simulink library "Normalization"  (R2014b)
settings: Solver=ode45  StartTime=0.0  StopTime=10.0  RelTol=1e-3
libraries: DivisionVectorScalar x1
settings Model: Creator=Hp  LastModifiedBy=Hp

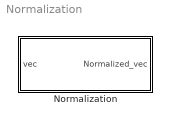
== system Normalization ==
  Normalization : Subsystem

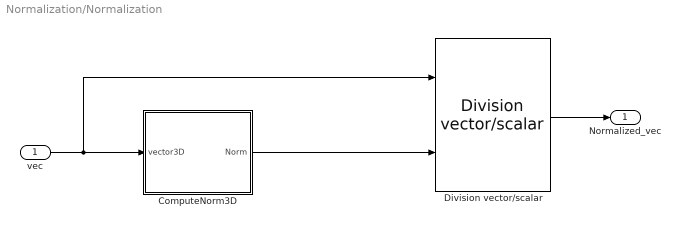
== system Normalization/Normalization ==
  vec : Inport
  ComputeNorm3D : Subsystem
  Division vector/scalar : DivisionVectorScalar/Division vector//scalar
  Normalized_vec : Outport
  wires:
  vec/1 -> Division vector/scalar/1, ComputeNorm3D/1(vector3D)
  Division vector/scalar/1 -> Normalized_vec/1
  ComputeNorm3D/1(Norm) -> Division vector/scalar/2

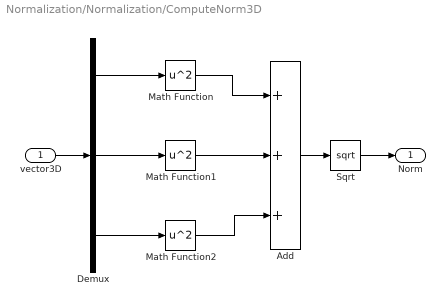
== system Normalization/Normalization/ComputeNorm3D ==
  vector3D : Inport
  Add : Sum  Inputs=+++
  Demux : Demux  Outputs=3
  Math Function : Math  Operator=square  SaturateOnIntegerOverflow=on
  Math Function1 : Math  Operator=square  SaturateOnIntegerOverflow=on
  Math Function2 : Math  Operator=square  SaturateOnIntegerOverflow=on
  Sqrt : Sqrt  SaturateOnIntegerOverflow=on
  Norm : Outport
  wires:
  vector3D/1 -> Demux/1
  Sqrt/1 -> Norm/1
  Add/1 -> Sqrt/1
  Math Function1/1 -> Add/2
  Math Function2/1 -> Add/3
  Demux/1 -> Math Function/1
  Math Function/1 -> Add/1
  Demux/3 -> Math Function2/1
  Demux/2 -> Math Function1/1
